simulink model "mat_acc"  (Simulink 8.7)
settings: Solver=VariableStepDiscrete  StartTime=0.0  StopTime=Accelerator_A10_param.endTime  MaxStep=1  RelTol=1e-3
PreLoadFcn:
  | % Run the setup script when the model is opened
  | setup_mat_acc;
InitFcn:
  | % Run the setup script again just before the
  | % model is run, so that any updates made
  | % after opening are applied.
  | setup_mat_acc;
undefined symbols (not defined in the file or in its folder): AdvDSPBChannelOutDisplay, dpoly, dspba_ChannelInVis, dspba_ChannelOutVis, dspba_internal_get_channel_ports, evalAionMaskParam, latency, primtype, value
libraries: DSPBAPrim x1114, DSPBAAvalonST x8, DSPBABase x5, DSPBAControl x2
(part 2 of 5)

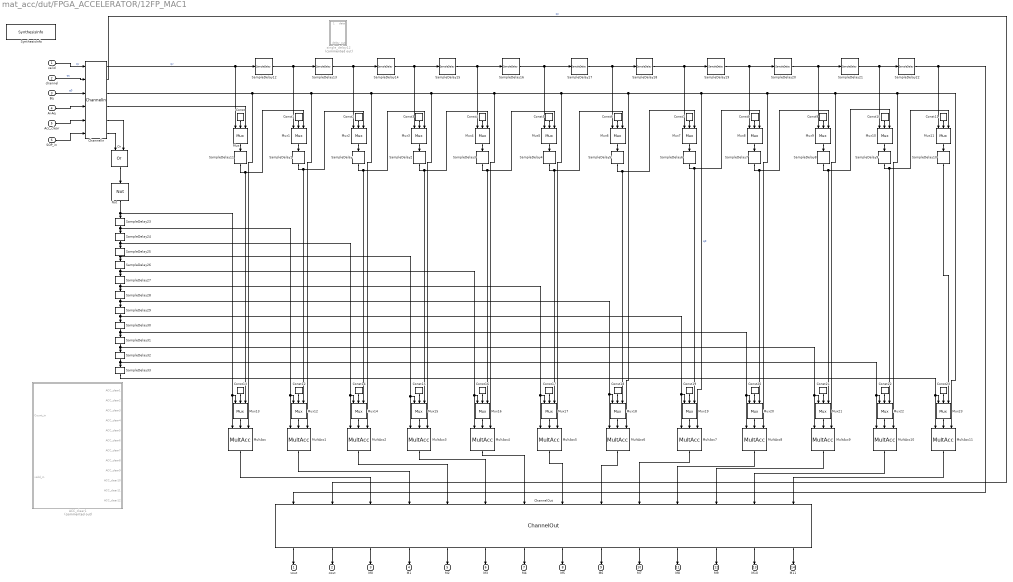
== system mat_acc/dut/FPGA_ACCELERATOR/12FP_MAC1 ==
  valid : Inport
  channel : Inport  Port=2
  Bq : Inport  Port=3
  Ai-Aq : Inport  Port=4
  Acc_clear : Inport  Port=5
  SOP_in : Inport  Port=6
  ACC_clear1 : Subsystem  Commented=on
  ChannelIn : DSPBAPrim/ChannelIn  primtype=channelin  nInputs=dspba_internal_get_channel_ports(gcb)  nOutputs=dspba_internal_get_channel_ports(gcb)  omode=Inherit via internal rule  otype=sfix(16)  scale=2^-15  rndmethod=Unbiased  factor=1  satmethod=Symmetric  shift_vec=[0 1 2 -1]  value=4  inPortNames=['v'; 'c'; '0'; '1'; '2'; '3'; '4'; '5'; '6'; '7'; '8'; '9'; 'A'; 'B'; 'D'; 'E'; 'F'; 'G'; 'H'; 'I'; 'J'; 'K'; 'L'; 'M'; 'N'; 'O'; 'P'; 'Q'; 'R'; 'S'; 'T'; 'U'; 'W'; 'X'; 'Y'; 'Z']  outPortNames=['v'; 'c'; '0'; '1'; '2'; '3'; '4'; '5'; '6'; '7'; '8'; '9'; 'A'; 'B'; 'D'; 'E'; 'F'; 'G'; 'H'; 'I'; 'J'; 'K'; 'L'; 'M'; 'N'; 'O'; 'P'; 'Q'; 'R'; 'S'; 'T'; 'U'; 'W'; 'X'; 'Y'; 'Z']  dspbaimage=dspba_prim.jpg  text=fprintf('In');  style=Optimised  dataSignals=4  foldingEnabled=off  channels=1  sampleRate=200  packetBeginPresent=off  packetBeginEnabled=off  visibilities=dspba_ChannelInVis(gcb)  latencyCorrection=0  version=20141013
  ChannelOut : DSPBAPrim/ChannelOut  primtype=channelout  nInputs=dspba_internal_get_channel_ports(gcb)  nOutputs=dspba_internal_get_channel_ports(gcb)  omode=Inherit via internal rule  otype=sfix(16)  scale=2^-15  rndmethod=Unbiased  factor=1  satmethod=Symmetric  shift_vec=[0 1 2 -1]  value=12  inPortNames=['v'; 'c'; '0'; '1'; '2'; '3'; '4'; '5'; '6'; '7'; '8'; '9'; 'A'; 'B'; 'D'; 'E'; 'F'; 'G'; 'H'; 'I'; 'J'; 'K'; 'L'; 'M'; 'N'; 'O'; 'P'; 'Q'; 'R'; 'S'; 'T'; 'U'; 'W'; 'X'; 'Y'; 'Z']  outPortNames=['v'; 'c'; '0'; '1'; '2'; '3'; '4'; '5'; '6'; '7'; '8'; '9'; 'A'; 'B'; 'D'; 'E'; 'F'; 'G'; 'H'; 'I'; 'J'; 'K'; 'L'; 'M'; 'N'; 'O'; 'P'; 'Q'; 'R'; 'S'; 'T'; 'U'; 'W'; 'X'; 'Y'; 'Z']  dspbaimage=dspba_prim.jpg  text=fprintf('Out%s', AdvDSPBChannelOutDisplay(latency));  style=Optimised  dataSignals=12  foldingEnabled=off  channels=1  sampleRate=200  packetBeginPresent=off  packetBeginEnabled=off  visibilities=dspba_ChannelOutVis(gcb)  latency=7  latencyCorrection=0  version=20141013
  Const{,1..23} (24 alike) : DSPBAPrim/Const  primtype=const  nInputs=0  nOutputs=1  omode=single  otype=sfix(16)  scale=2^-15  rndmethod=Unbiased  factor=1  satmethod=Symmetric  shift_vec=[0 1 2 -1]  value=0  inPortNames=['+'; '+';]  outPortNames=[' ']  dspbaimage=dspba_prim.jpg  text=fprintf('%s', num2str(value));  style=Optimised  visibilities=8 + 1024  floatPrecision=float32_m23  version=20120820
  MultAcc{,1..11} (12 alike) : DSPBAPrim/MultAcc  primtype=multaccfunc  nInputs=3  nOutputs=1  omode=Inherit via internal rule  otype=sfix(16)  scale=2^-15  rndmethod=Unbiased  factor=1  satmethod=Symmetric  shift_vec=[0 1 2 -1]  value=0  inPortNames="[ 'acc'; 'x  '; 'y  ']"  outPortNames=[]  dspbaimage=dspba_prim_float.jpg  text=disp('multAcc');  style=Optimised  visibilities=8+2^17  functionExpr=fpMultAcc  advOptions=[]  version=20121130
  Mux{,1..23} (24 alike) : DSPBAPrim/Mux  primtype=mux  nInputs=evalAionMaskParam(gcb,'value',1)+1  nOutputs=1  omode=Inherit via internal rule  otype=sfix(16)  scale=2^-15  rndmethod=Unbiased  factor=1  satmethod=Symmetric  shift_vec=[0 1 2 -1]  value=2  inPortNames=['s '; 'd0'; 'd1'; 'd2'; 'd3'; 'd4'; 'd5'; 'd6'; 'd7'; 'd8'; 'd9';]  outPortNames=[' ']  dspbaimage=dspba_prim.jpg  text=fprintf('%s', primtype);  style=Optimised  visibilities=1032  version=20131025
  Not : DSPBAPrim/Not  primtype=not  nInputs=1  nOutputs=1  omode=Inherit via internal rule  otype=sfix(16)  scale=2^-15  rndmethod=Unbiased  factor=1  satmethod=Symmetric  shift_vec=[0 1 2 -1]  value=0  inPortNames=[' '; ' ';]  outPortNames=[' ']  dspbaimage=dspba_prim.jpg  text=fprintf('~');  style=Optimised  visibilities=8  version=20090407
  Or : DSPBAPrim/Or  primtype=or  nInputs=2  nOutputs=1  omode=Inherit via internal rule  otype=sfix(16)  scale=2^-15  rndmethod=Unbiased  factor=1  satmethod=Symmetric  shift_vec=[0 1 2 -1]  value=0  inPortNames=[' '; ' '; ' '; ' '; ' '; ' '; ' '; ' '; ' '; ' '; ' '; ' '; ' '; ' '; ' '; ' '; ]  outPortNames=[' ']  dspbaimage=dspba_prim.jpg  text=fprintf('|');  style=Optimised  visibilities=8+2  version=20090407
  SampleDelay{,1..33} (34 alike) : DSPBAPrim/SampleDelay  primtype=sampdelay  nInputs=1  nOutputs=1  omode=Inherit via internal rule  otype=sfix(16)  scale=2^-15  rndmethod=Unbiased  factor=1  satmethod=Symmetric  shift_vec=[0 1 2 -1]  value=1  inPortNames=[' '; ' ';]  outPortNames=[' ']  dspbaimage=dspba_prim.jpg  text=dpoly(1, eye(1,value+1), 'z')  style=Optimised  visibilities=8 + 1024 + 2^17 + 2^18  flexible=off  slackgroup=0  augmented=0  version=20090407  advOptions=[]
  SynthesisInfo : DSPBAPrim/SynthesisInfo  primtype=synthinfo  nInputs=0  nOutputs=0  omode=Inherit via internal rule  otype=sfix(16)  scale=2^-15  rndmethod=Truncate  factor=1  satmethod=Symmetric  shift_vec=[0 1 2 -1]  value=99  inPortNames=[' '; ' ';]  outPortNames=[' ']  dspbaimage=dspba_prim_ctrl.jpg  text=fprintf('Style=%s', style);  style=Scheduled  visibilities=2^15+2^17+2^18+2^19  constraintInUse=on  constraintRelation==  constraintLimit=7  bitAccurate=off  version=20150220
  single_delay12 : Subsystem  Commented=on
  vout : Outport
  cout : Outport  Port=2
  M0 : Outport  Port=3
  M1 : Outport  Port=4
  M2 : Outport  Port=5
  M3 : Outport  Port=6
  M4 : Outport  Port=7
  M5 : Outport  Port=8
  M6 : Outport  Port=9
  M7 : Outport  Port=10
  M8 : Outport  Port=11
  M9 : Outport  Port=12
  M10 : Outport  Port=13
  M11 : Outport  Port=14
  wires:
  Mux23/1 -> MultAcc11/2
  Const23/1 -> Mux23/2
  Mux22/1 -> MultAcc10/2
  Const22/1 -> Mux22/2
  Mux21/1 -> MultAcc9/2
  Const21/1 -> Mux21/2
  Mux20/1 -> MultAcc8/2
  Const20/1 -> Mux20/2
  Mux19/1 -> MultAcc7/2
  Const19/1 -> Mux19/2
  Mux18/1 -> MultAcc6/2
  Const18/1 -> Mux18/2
  Mux17/1 -> MultAcc5/2
  Const17/1 -> Mux17/2
  Mux16/1 -> MultAcc4/2
  Const16/1 -> Mux16/2
  Mux15/1 -> MultAcc3/2
  Const15/1 -> Mux15/2
  Mux14/1 -> MultAcc2/2
  Const14/1 -> Mux14/2
  Mux12/1 -> MultAcc1/2
  Const12/1 -> Mux12/2
  Mux13/1 -> MultAcc/2
  Const13/1 -> Mux13/2
  Not/1 -> SampleDelay23/1, Mux13/1, MultAcc/1
  SampleDelay11/1 -> Mux1/3, Mux13/3
  Mux/1 -> SampleDelay11/1
  SampleDelay33/1 -> Mux23/1, MultAcc11/1
  SampleDelay32/1 -> SampleDelay33/1, MultAcc10/1, Mux22/1
  SampleDelay31/1 -> SampleDelay32/1, Mux21/1, MultAcc9/1
  SampleDelay30/1 -> SampleDelay31/1, MultAcc8/1, Mux20/1
  SampleDelay29/1 -> SampleDelay30/1, Mux19/1, MultAcc7/1
  SampleDelay28/1 -> SampleDelay29/1, Mux18/1, MultAcc6/1
  SampleDelay27/1 -> SampleDelay28/1, Mux17/1, MultAcc5/1
  SampleDelay26/1 -> SampleDelay27/1, Mux16/1, MultAcc4/1
  SampleDelay25/1 -> SampleDelay26/1, Mux15/1, MultAcc3/1
  SampleDelay24/1 -> SampleDelay25/1, Mux14/1, MultAcc2/1
  SampleDelay23/1 -> SampleDelay24/1, MultAcc1/1, Mux12/1
  SampleDelay22/1 -> Mux11/1, ChannelOut/1
  SampleDelay21/1 -> Mux10/1, SampleDelay22/1
  SampleDelay20/1 -> Mux9/1, SampleDelay21/1
  SampleDelay19/1 -> Mux8/1, SampleDelay20/1
  SampleDelay18/1 -> Mux7/1, SampleDelay19/1
  SampleDelay17/1 -> Mux6/1, SampleDelay18/1
  SampleDelay16/1 -> Mux5/1, SampleDelay17/1
  SampleDelay15/1 -> Mux4/1, SampleDelay16/1
  SampleDelay14/1 -> Mux3/1, SampleDelay15/1
  SampleDelay13/1 -> Mux2/1, SampleDelay14/1
  SampleDelay12/1 -> Mux1/1, SampleDelay13/1
  ChannelIn/6 -> Or/1
  SOP_in/1 -> ChannelIn/6
  ChannelIn/5 -> Or/2
  ChannelIn/1 -> Mux/1, SampleDelay12/1  "qv"
  SampleDelay10/1 -> Mux23/3
  SampleDelay9/1 -> Mux11/3, Mux22/3
  SampleDelay8/1 -> Mux10/3, Mux21/3
  SampleDelay7/1 -> Mux9/3, Mux20/3
  SampleDelay6/1 -> Mux8/3, Mux19/3
  SampleDelay5/1 -> Mux7/3, Mux18/3
  SampleDelay4/1 -> Mux6/3, Mux17/3
  SampleDelay3/1 -> Mux5/3, Mux16/3
  SampleDelay2/1 -> Mux4/3, Mux15/3
  SampleDelay1/1 -> Mux2/3, Mux12/3
  SampleDelay/1 -> Mux3/3, Mux14/3
  Const11/1 -> Mux11/2
  Const10/1 -> Mux10/2
  Const9/1 -> Mux9/2
  Const8/1 -> Mux8/2
  Const7/1 -> Mux7/2
  Const6/1 -> Mux6/2
  Const5/1 -> Mux5/2
  Const4/1 -> Mux4/2
  Const3/1 -> Mux3/2
  Const2/1 -> Mux2/2
  Const1/1 -> Mux1/2
  Const/1 -> Mux/2
  ChannelIn/2 -> ChannelOut/2  "qc"
  MultAcc11/1 -> ChannelOut/14
  MultAcc10/1 -> ChannelOut/13
  MultAcc9/1 -> ChannelOut/12
  MultAcc8/1 -> ChannelOut/11
  MultAcc7/1 -> ChannelOut/10
  MultAcc6/1 -> ChannelOut/9
  MultAcc5/1 -> ChannelOut/8
  MultAcc4/1 -> ChannelOut/7
  MultAcc3/1 -> ChannelOut/6
  MultAcc2/1 -> ChannelOut/5
  MultAcc1/1 -> ChannelOut/4
  MultAcc/1 -> ChannelOut/3
  ChannelOut/14 -> M11/1
  ChannelOut/13 -> M10/1
  ChannelOut/12 -> M9/1
  ChannelOut/11 -> M8/1
  ChannelOut/10 -> M7/1
  ChannelOut/9 -> M6/1
  ChannelOut/8 -> M5/1
  ChannelOut/7 -> M4/1
  ChannelOut/6 -> M3/1
  ChannelOut/5 -> M2/1
  ChannelOut/4 -> M1/1
  ChannelOut/3 -> M0/1
  ChannelOut/2 -> cout/1
  ChannelOut/1 -> vout/1
  Acc_clear/1 -> ChannelIn/5
  Ai-Aq/1 -> ChannelIn/4
  Bq/1 -> ChannelIn/3  "q0"
  channel/1 -> ChannelIn/2  "qc"
  valid/1 -> ChannelIn/1  "qv"
  Or/1 -> Not/1
  ChannelIn/4 -> Mux/3
  ChannelIn/3 -> MultAcc/3, MultAcc1/3, MultAcc2/3, MultAcc3/3, MultAcc4/3, MultAcc5/3, MultAcc6/3, MultAcc7/3, MultAcc8/3, MultAcc9/3, MultAcc10/3, MultAcc11/3  "q0"
  Mux1/1 -> SampleDelay1/1
  Mux2/1 -> SampleDelay/1
  Mux3/1 -> SampleDelay2/1
  Mux4/1 -> SampleDelay3/1
  Mux5/1 -> SampleDelay4/1
  Mux6/1 -> SampleDelay5/1
  Mux7/1 -> SampleDelay6/1
  Mux8/1 -> SampleDelay7/1
  Mux9/1 -> SampleDelay8/1
  Mux10/1 -> SampleDelay9/1
  Mux11/1 -> SampleDelay10/1

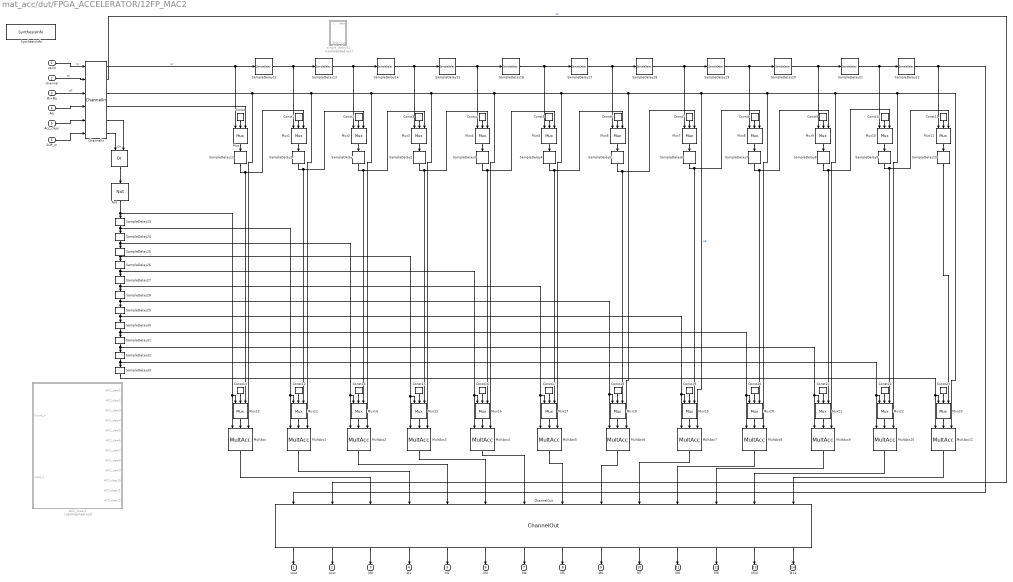
== system mat_acc/dut/FPGA_ACCELERATOR/12FP_MAC2 ==
  valid : Inport
  channel : Inport  Port=2
  Bi+Bq : Inport  Port=3
  Aq : Inport  Port=4
  Acc_clear : Inport  Port=5
  SOP_in : Inport  Port=6
  ACC_clear1 : Subsystem  Commented=on
  ChannelIn : DSPBAPrim/ChannelIn  primtype=channelin  nInputs=dspba_internal_get_channel_ports(gcb)  nOutputs=dspba_internal_get_channel_ports(gcb)  omode=Inherit via internal rule  otype=sfix(16)  scale=2^-15  rndmethod=Unbiased  factor=1  satmethod=Symmetric  shift_vec=[0 1 2 -1]  value=4  inPortNames=['v'; 'c'; '0'; '1'; '2'; '3'; '4'; '5'; '6'; '7'; '8'; '9'; 'A'; 'B'; 'D'; 'E'; 'F'; 'G'; 'H'; 'I'; 'J'; 'K'; 'L'; 'M'; 'N'; 'O'; 'P'; 'Q'; 'R'; 'S'; 'T'; 'U'; 'W'; 'X'; 'Y'; 'Z']  outPortNames=['v'; 'c'; '0'; '1'; '2'; '3'; '4'; '5'; '6'; '7'; '8'; '9'; 'A'; 'B'; 'D'; 'E'; 'F'; 'G'; 'H'; 'I'; 'J'; 'K'; 'L'; 'M'; 'N'; 'O'; 'P'; 'Q'; 'R'; 'S'; 'T'; 'U'; 'W'; 'X'; 'Y'; 'Z']  dspbaimage=dspba_prim.jpg  text=fprintf('In');  style=Optimised  dataSignals=4  foldingEnabled=off  channels=1  sampleRate=200  packetBeginPresent=off  packetBeginEnabled=off  visibilities=dspba_ChannelInVis(gcb)  latencyCorrection=0  version=20141013
  ChannelOut : DSPBAPrim/ChannelOut  primtype=channelout  nInputs=dspba_internal_get_channel_ports(gcb)  nOutputs=dspba_internal_get_channel_ports(gcb)  omode=Inherit via internal rule  otype=sfix(16)  scale=2^-15  rndmethod=Unbiased  factor=1  satmethod=Symmetric  shift_vec=[0 1 2 -1]  value=12  inPortNames=['v'; 'c'; '0'; '1'; '2'; '3'; '4'; '5'; '6'; '7'; '8'; '9'; 'A'; 'B'; 'D'; 'E'; 'F'; 'G'; 'H'; 'I'; 'J'; 'K'; 'L'; 'M'; 'N'; 'O'; 'P'; 'Q'; 'R'; 'S'; 'T'; 'U'; 'W'; 'X'; 'Y'; 'Z']  outPortNames=['v'; 'c'; '0'; '1'; '2'; '3'; '4'; '5'; '6'; '7'; '8'; '9'; 'A'; 'B'; 'D'; 'E'; 'F'; 'G'; 'H'; 'I'; 'J'; 'K'; 'L'; 'M'; 'N'; 'O'; 'P'; 'Q'; 'R'; 'S'; 'T'; 'U'; 'W'; 'X'; 'Y'; 'Z']  dspbaimage=dspba_prim.jpg  text=fprintf('Out%s', AdvDSPBChannelOutDisplay(latency));  style=Optimised  dataSignals=12  foldingEnabled=off  channels=1  sampleRate=200  packetBeginPresent=off  packetBeginEnabled=off  visibilities=dspba_ChannelOutVis(gcb)  latency=7  latencyCorrection=0  version=20141013
  Const{,1..23} (24 alike) : DSPBAPrim/Const  primtype=const  nInputs=0  nOutputs=1  omode=single  otype=sfix(16)  scale=2^-15  rndmethod=Unbiased  factor=1  satmethod=Symmetric  shift_vec=[0 1 2 -1]  value=0  inPortNames=['+'; '+';]  outPortNames=[' ']  dspbaimage=dspba_prim.jpg  text=fprintf('%s', num2str(value));  style=Optimised  visibilities=8 + 1024  floatPrecision=float32_m23  version=20120820
  MultAcc{,1..11} (12 alike) : DSPBAPrim/MultAcc  primtype=multaccfunc  nInputs=3  nOutputs=1  omode=Inherit via internal rule  otype=sfix(16)  scale=2^-15  rndmethod=Unbiased  factor=1  satmethod=Symmetric  shift_vec=[0 1 2 -1]  value=0  inPortNames="[ 'acc'; 'x  '; 'y  ']"  outPortNames=[]  dspbaimage=dspba_prim_float.jpg  text=disp('multAcc');  style=Optimised  visibilities=8+2^17  functionExpr=fpMultAcc  advOptions=[]  version=20121130
  Mux{,1..23} (24 alike) : DSPBAPrim/Mux  primtype=mux  nInputs=evalAionMaskParam(gcb,'value',1)+1  nOutputs=1  omode=Inherit via internal rule  otype=sfix(16)  scale=2^-15  rndmethod=Unbiased  factor=1  satmethod=Symmetric  shift_vec=[0 1 2 -1]  value=2  inPortNames=['s '; 'd0'; 'd1'; 'd2'; 'd3'; 'd4'; 'd5'; 'd6'; 'd7'; 'd8'; 'd9';]  outPortNames=[' ']  dspbaimage=dspba_prim.jpg  text=fprintf('%s', primtype);  style=Optimised  visibilities=1032  version=20131025
  Not : DSPBAPrim/Not  primtype=not  nInputs=1  nOutputs=1  omode=Inherit via internal rule  otype=sfix(16)  scale=2^-15  rndmethod=Unbiased  factor=1  satmethod=Symmetric  shift_vec=[0 1 2 -1]  value=0  inPortNames=[' '; ' ';]  outPortNames=[' ']  dspbaimage=dspba_prim.jpg  text=fprintf('~');  style=Optimised  visibilities=8  version=20090407
  Or : DSPBAPrim/Or  primtype=or  nInputs=2  nOutputs=1  omode=Inherit via internal rule  otype=sfix(16)  scale=2^-15  rndmethod=Unbiased  factor=1  satmethod=Symmetric  shift_vec=[0 1 2 -1]  value=0  inPortNames=[' '; ' '; ' '; ' '; ' '; ' '; ' '; ' '; ' '; ' '; ' '; ' '; ' '; ' '; ' '; ' '; ]  outPortNames=[' ']  dspbaimage=dspba_prim.jpg  text=fprintf('|');  style=Optimised  visibilities=8+2  version=20090407
  SampleDelay{,1..33} (34 alike) : DSPBAPrim/SampleDelay  primtype=sampdelay  nInputs=1  nOutputs=1  omode=Inherit via internal rule  otype=sfix(16)  scale=2^-15  rndmethod=Unbiased  factor=1  satmethod=Symmetric  shift_vec=[0 1 2 -1]  value=1  inPortNames=[' '; ' ';]  outPortNames=[' ']  dspbaimage=dspba_prim.jpg  text=dpoly(1, eye(1,value+1), 'z')  style=Optimised  visibilities=8 + 1024 + 2^17 + 2^18  flexible=off  slackgroup=0  augmented=0  version=20090407  advOptions=[]
  SynthesisInfo : DSPBAPrim/SynthesisInfo  primtype=synthinfo  nInputs=0  nOutputs=0  omode=Inherit via internal rule  otype=sfix(16)  scale=2^-15  rndmethod=Truncate  factor=1  satmethod=Symmetric  shift_vec=[0 1 2 -1]  value=99  inPortNames=[' '; ' ';]  outPortNames=[' ']  dspbaimage=dspba_prim_ctrl.jpg  text=fprintf('Style=%s', style);  style=Scheduled  visibilities=2^15+2^17+2^18+2^19  constraintInUse=on  constraintRelation==  constraintLimit=7  bitAccurate=off  version=20150220
  single_delay12 : Subsystem  Commented=on
  vout : Outport
  cout : Outport  Port=2
  M0 : Outport  Port=3
  M1 : Outport  Port=4
  M2 : Outport  Port=5
  M3 : Outport  Port=6
  M4 : Outport  Port=7
  M5 : Outport  Port=8
  M6 : Outport  Port=9
  M7 : Outport  Port=10
  M8 : Outport  Port=11
  M9 : Outport  Port=12
  M10 : Outport  Port=13
  M11 : Outport  Port=14
  wires:
  Mux11/1 -> SampleDelay10/1
  Mux10/1 -> SampleDelay9/1
  Mux9/1 -> SampleDelay8/1
  Mux8/1 -> SampleDelay7/1
  Mux7/1 -> SampleDelay6/1
  Mux6/1 -> SampleDelay5/1
  Mux5/1 -> SampleDelay4/1
  Mux4/1 -> SampleDelay3/1
  Mux3/1 -> SampleDelay2/1
  Mux2/1 -> SampleDelay/1
  Mux1/1 -> SampleDelay1/1
  ChannelIn/3 -> MultAcc11/3, MultAcc10/3, MultAcc9/3, MultAcc8/3, MultAcc7/3, MultAcc6/3, MultAcc5/3, MultAcc4/3, MultAcc3/3, MultAcc2/3, MultAcc1/3, MultAcc/3  "q0"
  ChannelIn/4 -> Mux/3
  Or/1 -> Not/1
  valid/1 -> ChannelIn/1  "qv"
  channel/1 -> ChannelIn/2  "qc"
  Bi+Bq/1 -> ChannelIn/3  "q0"
  Aq/1 -> ChannelIn/4
  Acc_clear/1 -> ChannelIn/5
  ChannelOut/1 -> vout/1
  ChannelOut/2 -> cout/1
  ChannelOut/3 -> M0/1
  ChannelOut/4 -> M1/1
  ChannelOut/5 -> M2/1
  ChannelOut/6 -> M3/1
  ChannelOut/7 -> M4/1
  ChannelOut/8 -> M5/1
  ChannelOut/9 -> M6/1
  ChannelOut/10 -> M7/1
  ChannelOut/11 -> M8/1
  ChannelOut/12 -> M9/1
  ChannelOut/13 -> M10/1
  ChannelOut/14 -> M11/1
  MultAcc/1 -> ChannelOut/3
  MultAcc1/1 -> ChannelOut/4
  MultAcc2/1 -> ChannelOut/5
  MultAcc3/1 -> ChannelOut/6
  MultAcc4/1 -> ChannelOut/7
  MultAcc5/1 -> ChannelOut/8
  MultAcc6/1 -> ChannelOut/9
  MultAcc7/1 -> ChannelOut/10
  MultAcc8/1 -> ChannelOut/11
  MultAcc9/1 -> ChannelOut/12
  MultAcc10/1 -> ChannelOut/13
  MultAcc11/1 -> ChannelOut/14
  ChannelIn/2 -> ChannelOut/2  "qc"
  Const/1 -> Mux/2
  Const1/1 -> Mux1/2
  Const2/1 -> Mux2/2
  Const3/1 -> Mux3/2
  Const4/1 -> Mux4/2
  Const5/1 -> Mux5/2
  Const6/1 -> Mux6/2
  Const7/1 -> Mux7/2
  Const8/1 -> Mux8/2
  Const9/1 -> Mux9/2
  Const10/1 -> Mux10/2
  Const11/1 -> Mux11/2
  SampleDelay/1 -> Mux14/3, Mux3/3
  SampleDelay1/1 -> Mux12/3, Mux2/3
  SampleDelay2/1 -> Mux15/3, Mux4/3
  SampleDelay3/1 -> Mux16/3, Mux5/3
  SampleDelay4/1 -> Mux17/3, Mux6/3
  SampleDelay5/1 -> Mux18/3, Mux7/3
  SampleDelay6/1 -> Mux19/3, Mux8/3
  SampleDelay7/1 -> Mux20/3, Mux9/3
  SampleDelay8/1 -> Mux21/3, Mux10/3
  SampleDelay9/1 -> Mux22/3, Mux11/3
  SampleDelay10/1 -> Mux23/3
  ChannelIn/1 -> SampleDelay12/1, Mux/1  "qv"
  ChannelIn/5 -> Or/2
  SOP_in/1 -> ChannelIn/6
  ChannelIn/6 -> Or/1
  SampleDelay12/1 -> SampleDelay13/1, Mux1/1
  SampleDelay13/1 -> SampleDelay14/1, Mux2/1
  SampleDelay14/1 -> SampleDelay15/1, Mux3/1
  SampleDelay15/1 -> SampleDelay16/1, Mux4/1
  SampleDelay16/1 -> SampleDelay17/1, Mux5/1
  SampleDelay17/1 -> SampleDelay18/1, Mux6/1
  SampleDelay18/1 -> SampleDelay19/1, Mux7/1
  SampleDelay19/1 -> SampleDelay20/1, Mux8/1
  SampleDelay20/1 -> SampleDelay21/1, Mux9/1
  SampleDelay21/1 -> SampleDelay22/1, Mux10/1
  SampleDelay22/1 -> ChannelOut/1, Mux11/1
  SampleDelay23/1 -> Mux12/1, MultAcc1/1, SampleDelay24/1
  SampleDelay24/1 -> MultAcc2/1, Mux14/1, SampleDelay25/1
  SampleDelay25/1 -> MultAcc3/1, Mux15/1, SampleDelay26/1
  SampleDelay26/1 -> MultAcc4/1, Mux16/1, SampleDelay27/1
  SampleDelay27/1 -> MultAcc5/1, Mux17/1, SampleDelay28/1
  SampleDelay28/1 -> MultAcc6/1, Mux18/1, SampleDelay29/1
  SampleDelay29/1 -> MultAcc7/1, Mux19/1, SampleDelay30/1
  SampleDelay30/1 -> Mux20/1, MultAcc8/1, SampleDelay31/1
  SampleDelay31/1 -> MultAcc9/1, Mux21/1, SampleDelay32/1
  SampleDelay32/1 -> Mux22/1, MultAcc10/1, SampleDelay33/1
  SampleDelay33/1 -> MultAcc11/1, Mux23/1
  Mux/1 -> SampleDelay11/1
  SampleDelay11/1 -> Mux13/3, Mux1/3
  Not/1 -> MultAcc/1, Mux13/1, SampleDelay23/1
  Const13/1 -> Mux13/2
  Mux13/1 -> MultAcc/2
  Const12/1 -> Mux12/2
  Mux12/1 -> MultAcc1/2
  Const14/1 -> Mux14/2
  Mux14/1 -> MultAcc2/2
  Const15/1 -> Mux15/2
  Mux15/1 -> MultAcc3/2
  Const16/1 -> Mux16/2
  Mux16/1 -> MultAcc4/2
  Const17/1 -> Mux17/2
  Mux17/1 -> MultAcc5/2
  Const18/1 -> Mux18/2
  Mux18/1 -> MultAcc6/2
  Const19/1 -> Mux19/2
  Mux19/1 -> MultAcc7/2
  Const20/1 -> Mux20/2
  Mux20/1 -> MultAcc8/2
  Const21/1 -> Mux21/2
  Mux21/1 -> MultAcc9/2
  Const22/1 -> Mux22/2
  Mux22/1 -> MultAcc10/2
  Const23/1 -> Mux23/2
  Mux23/1 -> MultAcc11/2

== system mat_acc/dut/FPGA_ACCELERATOR/12FP_MUX ==
  Valid : Inport
  Channel : Inport  Port=2
  I0 : Inport  Port=3
  I1 : Inport  Port=4
  I2 : Inport  Port=5
  I3 : Inport  Port=6
  I4 : Inport  Port=7
  I5 : Inport  Port=8
  I6 : Inport  Port=9
  I7 : Inport  Port=10
  I8 : Inport  Port=11
  I9 : Inport  Port=12
  I10 : Inport  Port=13
  I11 : Inport  Port=14
  MUX_select : Inport  Port=15
  ChannelIn : DSPBAPrim/ChannelIn  primtype=channelin  nInputs=dspba_internal_get_channel_ports(gcb)  nOutputs=dspba_internal_get_channel_ports(gcb)  omode=Inherit via internal rule  otype=sfix(16)  scale=2^-15  rndmethod=Unbiased  factor=1  satmethod=Symmetric  shift_vec=[0 1 2 -1]  value=13  inPortNames=['v'; 'c'; '0'; '1'; '2'; '3'; '4'; '5'; '6'; '7'; '8'; '9'; 'A'; 'B'; 'D'; 'E'; 'F'; 'G'; 'H'; 'I'; 'J'; 'K'; 'L'; 'M'; 'N'; 'O'; 'P'; 'Q'; 'R'; 'S'; 'T'; 'U'; 'W'; 'X'; 'Y'; 'Z']  outPortNames=['v'; 'c'; '0'; '1'; '2'; '3'; '4'; '5'; '6'; '7'; '8'; '9'; 'A'; 'B'; 'D'; 'E'; 'F'; 'G'; 'H'; 'I'; 'J'; 'K'; 'L'; 'M'; 'N'; 'O'; 'P'; 'Q'; 'R'; 'S'; 'T'; 'U'; 'W'; 'X'; 'Y'; 'Z']  dspbaimage=dspba_prim.jpg  text=fprintf('In');  style=Optimised  dataSignals=13  foldingEnabled=off  channels=1  sampleRate=200  packetBeginPresent=off  packetBeginEnabled=off  visibilities=dspba_ChannelInVis(gcb)  latencyCorrection=0  version=20141013
  ChannelOut : DSPBAPrim/ChannelOut  primtype=channelout  nInputs=dspba_internal_get_channel_ports(gcb)  nOutputs=dspba_internal_get_channel_ports(gcb)  omode=Inherit via internal rule  otype=sfix(16)  scale=2^-15  rndmethod=Unbiased  factor=1  satmethod=Symmetric  shift_vec=[0 1 2 -1]  value=1  inPortNames=['v'; 'c'; '0'; '1'; '2'; '3'; '4'; '5'; '6'; '7'; '8'; '9'; 'A'; 'B'; 'D'; 'E'; 'F'; 'G'; 'H'; 'I'; 'J'; 'K'; 'L'; 'M'; 'N'; 'O'; 'P'; 'Q'; 'R'; 'S'; 'T'; 'U'; 'W'; 'X'; 'Y'; 'Z']  outPortNames=['v'; 'c'; '0'; '1'; '2'; '3'; '4'; '5'; '6'; '7'; '8'; '9'; 'A'; 'B'; 'D'; 'E'; 'F'; 'G'; 'H'; 'I'; 'J'; 'K'; 'L'; 'M'; 'N'; 'O'; 'P'; 'Q'; 'R'; 'S'; 'T'; 'U'; 'W'; 'X'; 'Y'; 'Z']  dspbaimage=dspba_prim.jpg  text=fprintf('Out%s', AdvDSPBChannelOutDisplay(latency));  style=Optimised  dataSignals=1  foldingEnabled=off  channels=1  sampleRate=200  packetBeginPresent=off  packetBeginEnabled=off  visibilities=dspba_ChannelOutVis(gcb)  latency=2  latencyCorrection=0  version=20141013
  Const : DSPBAPrim/Const  primtype=const  nInputs=0  nOutputs=1  omode=single  otype=sfix(16)  scale=2^-15  rndmethod=Unbiased  factor=1  satmethod=Symmetric  shift_vec=[0 1 2 -1]  value=0  inPortNames=['+'; '+';]  outPortNames=[' ']  dspbaimage=dspba_prim.jpg  text=fprintf('%s', num2str(value));  style=Optimised  visibilities=8 + 1024  floatPrecision=float32_m23  version=20120820
  Mux real : DSPBAPrim/Mux  primtype=mux  nInputs=evalAionMaskParam(gcb,'value',1)+1  nOutputs=1  omode=Inherit via internal rule  otype=sfix(16)  scale=2^-15  rndmethod=Unbiased  factor=1  satmethod=Symmetric  shift_vec=[0 1 2 -1]  value=13  inPortNames=['s '; 'd0'; 'd1'; 'd2'; 'd3'; 'd4'; 'd5'; 'd6'; 'd7'; 'd8'; 'd9';]  outPortNames=[' ']  dspbaimage=dspba_prim.jpg  text=fprintf('%s', primtype);  style=Optimised  visibilities=1032  version=20131025
  SampleDelay : DSPBAPrim/SampleDelay  primtype=sampdelay  nInputs=1  nOutputs=1  omode=Inherit via internal rule  otype=sfix(16)  scale=2^-15  rndmethod=Unbiased  factor=1  satmethod=Symmetric  shift_vec=[0 1 2 -1]  value=5  inPortNames=[' '; ' ';]  outPortNames=[' ']  dspbaimage=dspba_prim.jpg  text=dpoly(1, eye(1,value+1), 'z')  style=Optimised  visibilities=8 + 1024 + 2^17 + 2^18  flexible=off  slackgroup=0  augmented=0  version=20090407  advOptions=[]
  SynthesisInfo : DSPBAPrim/SynthesisInfo  primtype=synthinfo  nInputs=0  nOutputs=0  omode=Inherit via internal rule  otype=sfix(16)  scale=2^-15  rndmethod=Truncate  factor=1  satmethod=Symmetric  shift_vec=[0 1 2 -1]  value=99  inPortNames=[' '; ' ';]  outPortNames=[' ']  dspbaimage=dspba_prim_ctrl.jpg  text=fprintf('Style=%s', style);  style=Scheduled  visibilities=2^15+2^17+2^18+2^19  constraintInUse=on  constraintRelation==  constraintLimit=2  bitAccurate=off  version=20150220
  vout : Outport
  cout : Outport  Port=2
  (Bi-Bq)*Ai : Outport  Port=3
  wires:
  ChannelIn/14 -> Mux real/14
  ChannelIn/13 -> Mux real/13
  ChannelIn/12 -> Mux real/12
  ChannelIn/11 -> Mux real/11
  ChannelIn/10 -> Mux real/10
  ChannelIn/9 -> Mux real/9
  ChannelIn/8 -> Mux real/8
  ChannelIn/7 -> Mux real/7
  ChannelIn/6 -> Mux real/6
  ChannelIn/5 -> Mux real/5
  ChannelIn/4 -> Mux real/4
  ChannelIn/3 -> Mux real/3
  ChannelIn/15 -> SampleDelay/1
  ChannelIn/2 -> ChannelOut/2
  Mux real/1 -> ChannelOut/3
  Const/1 -> Mux real/2
  Valid/1 -> ChannelIn/1
  Channel/1 -> ChannelIn/2
  I0/1 -> ChannelIn/3
  I1/1 -> ChannelIn/4
  I2/1 -> ChannelIn/5
  I3/1 -> ChannelIn/6
  I4/1 -> ChannelIn/7
  I5/1 -> ChannelIn/8
  I6/1 -> ChannelIn/9
  I7/1 -> ChannelIn/10
  I8/1 -> ChannelIn/11
  I9/1 -> ChannelIn/12
  I10/1 -> ChannelIn/13
  I11/1 -> ChannelIn/14
  MUX_select/1 -> ChannelIn/15
  ChannelOut/1 -> vout/1
  ChannelOut/2 -> cout/1
  ChannelOut/3 -> (Bi-Bq)*Ai/1
  SampleDelay/1 -> Mux real/1
  ChannelIn/1 -> ChannelOut/1

== system mat_acc/dut/FPGA_ACCELERATOR/12FP_MUX1 ==
  Valid : Inport
  Channel : Inport  Port=2
  I0 : Inport  Port=3
  I1 : Inport  Port=4
  I2 : Inport  Port=5
  I3 : Inport  Port=6
  I4 : Inport  Port=7
  I5 : Inport  Port=8
  I6 : Inport  Port=9
  I7 : Inport  Port=10
  I8 : Inport  Port=11
  I9 : Inport  Port=12
  I10 : Inport  Port=13
  I11 : Inport  Port=14
  MUX_select : Inport  Port=15
  ChannelIn : DSPBAPrim/ChannelIn  primtype=channelin  nInputs=dspba_internal_get_channel_ports(gcb)  nOutputs=dspba_internal_get_channel_ports(gcb)  omode=Inherit via internal rule  otype=sfix(16)  scale=2^-15  rndmethod=Unbiased  factor=1  satmethod=Symmetric  shift_vec=[0 1 2 -1]  value=13  inPortNames=['v'; 'c'; '0'; '1'; '2'; '3'; '4'; '5'; '6'; '7'; '8'; '9'; 'A'; 'B'; 'D'; 'E'; 'F'; 'G'; 'H'; 'I'; 'J'; 'K'; 'L'; 'M'; 'N'; 'O'; 'P'; 'Q'; 'R'; 'S'; 'T'; 'U'; 'W'; 'X'; 'Y'; 'Z']  outPortNames=['v'; 'c'; '0'; '1'; '2'; '3'; '4'; '5'; '6'; '7'; '8'; '9'; 'A'; 'B'; 'D'; 'E'; 'F'; 'G'; 'H'; 'I'; 'J'; 'K'; 'L'; 'M'; 'N'; 'O'; 'P'; 'Q'; 'R'; 'S'; 'T'; 'U'; 'W'; 'X'; 'Y'; 'Z']  dspbaimage=dspba_prim.jpg  text=fprintf('In');  style=Optimised  dataSignals=13  foldingEnabled=off  channels=1  sampleRate=200  packetBeginPresent=off  packetBeginEnabled=off  visibilities=dspba_ChannelInVis(gcb)  latencyCorrection=0  version=20141013
  ChannelOut : DSPBAPrim/ChannelOut  primtype=channelout  nInputs=dspba_internal_get_channel_ports(gcb)  nOutputs=dspba_internal_get_channel_ports(gcb)  omode=Inherit via internal rule  otype=sfix(16)  scale=2^-15  rndmethod=Unbiased  factor=1  satmethod=Symmetric  shift_vec=[0 1 2 -1]  value=1  inPortNames=['v'; 'c'; '0'; '1'; '2'; '3'; '4'; '5'; '6'; '7'; '8'; '9'; 'A'; 'B'; 'D'; 'E'; 'F'; 'G'; 'H'; 'I'; 'J'; 'K'; 'L'; 'M'; 'N'; 'O'; 'P'; 'Q'; 'R'; 'S'; 'T'; 'U'; 'W'; 'X'; 'Y'; 'Z']  outPortNames=['v'; 'c'; '0'; '1'; '2'; '3'; '4'; '5'; '6'; '7'; '8'; '9'; 'A'; 'B'; 'D'; 'E'; 'F'; 'G'; 'H'; 'I'; 'J'; 'K'; 'L'; 'M'; 'N'; 'O'; 'P'; 'Q'; 'R'; 'S'; 'T'; 'U'; 'W'; 'X'; 'Y'; 'Z']  dspbaimage=dspba_prim.jpg  text=fprintf('Out%s', AdvDSPBChannelOutDisplay(latency));  style=Optimised  dataSignals=1  foldingEnabled=off  channels=1  sampleRate=200  packetBeginPresent=off  packetBeginEnabled=off  visibilities=dspba_ChannelOutVis(gcb)  latency=2  latencyCorrection=0  version=20141013
  Const : DSPBAPrim/Const  primtype=const  nInputs=0  nOutputs=1  omode=single  otype=sfix(16)  scale=2^-15  rndmethod=Unbiased  factor=1  satmethod=Symmetric  shift_vec=[0 1 2 -1]  value=0  inPortNames=['+'; '+';]  outPortNames=[' ']  dspbaimage=dspba_prim.jpg  text=fprintf('%s', num2str(value));  style=Optimised  visibilities=8 + 1024  floatPrecision=float32_m23  version=20120820
  Mux real : DSPBAPrim/Mux  primtype=mux  nInputs=evalAionMaskParam(gcb,'value',1)+1  nOutputs=1  omode=Inherit via internal rule  otype=sfix(16)  scale=2^-15  rndmethod=Unbiased  factor=1  satmethod=Symmetric  shift_vec=[0 1 2 -1]  value=13  inPortNames=['s '; 'd0'; 'd1'; 'd2'; 'd3'; 'd4'; 'd5'; 'd6'; 'd7'; 'd8'; 'd9';]  outPortNames=[' ']  dspbaimage=dspba_prim.jpg  text=fprintf('%s', primtype);  style=Optimised  visibilities=1032  version=20131025
  SampleDelay : DSPBAPrim/SampleDelay  primtype=sampdelay  nInputs=1  nOutputs=1  omode=Inherit via internal rule  otype=sfix(16)  scale=2^-15  rndmethod=Unbiased  factor=1  satmethod=Symmetric  shift_vec=[0 1 2 -1]  value=5  inPortNames=[' '; ' ';]  outPortNames=[' ']  dspbaimage=dspba_prim.jpg  text=dpoly(1, eye(1,value+1), 'z')  style=Optimised  visibilities=8 + 1024 + 2^17 + 2^18  flexible=off  slackgroup=0  augmented=0  version=20090407  advOptions=[]
  SynthesisInfo : DSPBAPrim/SynthesisInfo  primtype=synthinfo  nInputs=0  nOutputs=0  omode=Inherit via internal rule  otype=sfix(16)  scale=2^-15  rndmethod=Truncate  factor=1  satmethod=Symmetric  shift_vec=[0 1 2 -1]  value=99  inPortNames=[' '; ' ';]  outPortNames=[' ']  dspbaimage=dspba_prim_ctrl.jpg  text=fprintf('Style=%s', style);  style=Scheduled  visibilities=2^15+2^17+2^18+2^19  constraintInUse=on  constraintRelation==  constraintLimit=2  bitAccurate=off  version=20150220
  vout : Outport
  cout : Outport  Port=2
  Bq*(Ai-Aq) : Outport  Port=3
  wires:
  ChannelOut/3 -> Bq*(Ai-Aq)/1
  ChannelOut/2 -> cout/1
  ChannelOut/1 -> vout/1
  MUX_select/1 -> ChannelIn/15
  I11/1 -> ChannelIn/14
  I10/1 -> ChannelIn/13
  I9/1 -> ChannelIn/12
  I8/1 -> ChannelIn/11
  I7/1 -> ChannelIn/10
  I6/1 -> ChannelIn/9
  I5/1 -> ChannelIn/8
  I4/1 -> ChannelIn/7
  I3/1 -> ChannelIn/6
  I2/1 -> ChannelIn/5
  I1/1 -> ChannelIn/4
  I0/1 -> ChannelIn/3
  Channel/1 -> ChannelIn/2
  Valid/1 -> ChannelIn/1
  Const/1 -> Mux real/2
  Mux real/1 -> ChannelOut/3
  ChannelIn/2 -> ChannelOut/2
  ChannelIn/1 -> ChannelOut/1
  ChannelIn/15 -> SampleDelay/1
  ChannelIn/3 -> Mux real/3
  ChannelIn/4 -> Mux real/4
  ChannelIn/5 -> Mux real/5
  ChannelIn/6 -> Mux real/6
  ChannelIn/7 -> Mux real/7
  ChannelIn/8 -> Mux real/8
  ChannelIn/9 -> Mux real/9
  ChannelIn/10 -> Mux real/10
  ChannelIn/11 -> Mux real/11
  ChannelIn/12 -> Mux real/12
  ChannelIn/13 -> Mux real/13
  ChannelIn/14 -> Mux real/14
  SampleDelay/1 -> Mux real/1

== system mat_acc/dut/FPGA_ACCELERATOR/12FP_MUX2 ==
  Valid : Inport
  Channel : Inport  Port=2
  I0 : Inport  Port=3
  I1 : Inport  Port=4
  I2 : Inport  Port=5
  I3 : Inport  Port=6
  I4 : Inport  Port=7
  I5 : Inport  Port=8
  I6 : Inport  Port=9
  I7 : Inport  Port=10
  I8 : Inport  Port=11
  I9 : Inport  Port=12
  I10 : Inport  Port=13
  I11 : Inport  Port=14
  MUX_select : Inport  Port=15
  ChannelIn : DSPBAPrim/ChannelIn  primtype=channelin  nInputs=dspba_internal_get_channel_ports(gcb)  nOutputs=dspba_internal_get_channel_ports(gcb)  omode=Inherit via internal rule  otype=sfix(16)  scale=2^-15  rndmethod=Unbiased  factor=1  satmethod=Symmetric  shift_vec=[0 1 2 -1]  value=13  inPortNames=['v'; 'c'; '0'; '1'; '2'; '3'; '4'; '5'; '6'; '7'; '8'; '9'; 'A'; 'B'; 'D'; 'E'; 'F'; 'G'; 'H'; 'I'; 'J'; 'K'; 'L'; 'M'; 'N'; 'O'; 'P'; 'Q'; 'R'; 'S'; 'T'; 'U'; 'W'; 'X'; 'Y'; 'Z']  outPortNames=['v'; 'c'; '0'; '1'; '2'; '3'; '4'; '5'; '6'; '7'; '8'; '9'; 'A'; 'B'; 'D'; 'E'; 'F'; 'G'; 'H'; 'I'; 'J'; 'K'; 'L'; 'M'; 'N'; 'O'; 'P'; 'Q'; 'R'; 'S'; 'T'; 'U'; 'W'; 'X'; 'Y'; 'Z']  dspbaimage=dspba_prim.jpg  text=fprintf('In');  style=Optimised  dataSignals=13  foldingEnabled=off  channels=1  sampleRate=200  packetBeginPresent=off  packetBeginEnabled=off  visibilities=dspba_ChannelInVis(gcb)  latencyCorrection=0  version=20141013
  ChannelOut : DSPBAPrim/ChannelOut  primtype=channelout  nInputs=dspba_internal_get_channel_ports(gcb)  nOutputs=dspba_internal_get_channel_ports(gcb)  omode=Inherit via internal rule  otype=sfix(16)  scale=2^-15  rndmethod=Unbiased  factor=1  satmethod=Symmetric  shift_vec=[0 1 2 -1]  value=1  inPortNames=['v'; 'c'; '0'; '1'; '2'; '3'; '4'; '5'; '6'; '7'; '8'; '9'; 'A'; 'B'; 'D'; 'E'; 'F'; 'G'; 'H'; 'I'; 'J'; 'K'; 'L'; 'M'; 'N'; 'O'; 'P'; 'Q'; 'R'; 'S'; 'T'; 'U'; 'W'; 'X'; 'Y'; 'Z']  outPortNames=['v'; 'c'; '0'; '1'; '2'; '3'; '4'; '5'; '6'; '7'; '8'; '9'; 'A'; 'B'; 'D'; 'E'; 'F'; 'G'; 'H'; 'I'; 'J'; 'K'; 'L'; 'M'; 'N'; 'O'; 'P'; 'Q'; 'R'; 'S'; 'T'; 'U'; 'W'; 'X'; 'Y'; 'Z']  dspbaimage=dspba_prim.jpg  text=fprintf('Out%s', AdvDSPBChannelOutDisplay(latency));  style=Optimised  dataSignals=1  foldingEnabled=off  channels=1  sampleRate=200  packetBeginPresent=off  packetBeginEnabled=off  visibilities=dspba_ChannelOutVis(gcb)  latency=2  latencyCorrection=0  version=20141013
  Const : DSPBAPrim/Const  primtype=const  nInputs=0  nOutputs=1  omode=single  otype=sfix(16)  scale=2^-15  rndmethod=Unbiased  factor=1  satmethod=Symmetric  shift_vec=[0 1 2 -1]  value=0  inPortNames=['+'; '+';]  outPortNames=[' ']  dspbaimage=dspba_prim.jpg  text=fprintf('%s', num2str(value));  style=Optimised  visibilities=8 + 1024  floatPrecision=float32_m23  version=20120820
  Mux real : DSPBAPrim/Mux  primtype=mux  nInputs=evalAionMaskParam(gcb,'value',1)+1  nOutputs=1  omode=Inherit via internal rule  otype=sfix(16)  scale=2^-15  rndmethod=Unbiased  factor=1  satmethod=Symmetric  shift_vec=[0 1 2 -1]  value=13  inPortNames=['s '; 'd0'; 'd1'; 'd2'; 'd3'; 'd4'; 'd5'; 'd6'; 'd7'; 'd8'; 'd9';]  outPortNames=[' ']  dspbaimage=dspba_prim.jpg  text=fprintf('%s', primtype);  style=Optimised  visibilities=1032  version=20131025
  SampleDelay : DSPBAPrim/SampleDelay  primtype=sampdelay  nInputs=1  nOutputs=1  omode=Inherit via internal rule  otype=sfix(16)  scale=2^-15  rndmethod=Unbiased  factor=1  satmethod=Symmetric  shift_vec=[0 1 2 -1]  value=5  inPortNames=[' '; ' ';]  outPortNames=[' ']  dspbaimage=dspba_prim.jpg  text=dpoly(1, eye(1,value+1), 'z')  style=Optimised  visibilities=8 + 1024 + 2^17 + 2^18  flexible=off  slackgroup=0  augmented=0  version=20090407  advOptions=[]
  SynthesisInfo : DSPBAPrim/SynthesisInfo  primtype=synthinfo  nInputs=0  nOutputs=0  omode=Inherit via internal rule  otype=sfix(16)  scale=2^-15  rndmethod=Truncate  factor=1  satmethod=Symmetric  shift_vec=[0 1 2 -1]  value=99  inPortNames=[' '; ' ';]  outPortNames=[' ']  dspbaimage=dspba_prim_ctrl.jpg  text=fprintf('Style=%s', style);  style=Scheduled  visibilities=2^15+2^17+2^18+2^19  constraintInUse=on  constraintRelation==  constraintLimit=2  bitAccurate=off  version=20150220
  vout : Outport
  cout : Outport  Port=2
  (Bi+Bq)*Aq : Outport  Port=3
  wires:
  ChannelIn/14 -> Mux real/14
  ChannelIn/13 -> Mux real/13
  ChannelIn/12 -> Mux real/12
  ChannelIn/11 -> Mux real/11
  ChannelIn/10 -> Mux real/10
  ChannelIn/9 -> Mux real/9
  ChannelIn/8 -> Mux real/8
  ChannelIn/7 -> Mux real/7
  ChannelIn/6 -> Mux real/6
  ChannelIn/5 -> Mux real/5
  ChannelIn/4 -> Mux real/4
  ChannelIn/3 -> Mux real/3
  ChannelIn/15 -> SampleDelay/1
  ChannelIn/1 -> ChannelOut/1
  ChannelIn/2 -> ChannelOut/2
  Mux real/1 -> ChannelOut/3
  Const/1 -> Mux real/2
  Valid/1 -> ChannelIn/1
  Channel/1 -> ChannelIn/2
  I0/1 -> ChannelIn/3
  I1/1 -> ChannelIn/4
  I2/1 -> ChannelIn/5
  I3/1 -> ChannelIn/6
  I4/1 -> ChannelIn/7
  I5/1 -> ChannelIn/8
  I6/1 -> ChannelIn/9
  I7/1 -> ChannelIn/10
  I8/1 -> ChannelIn/11
  I9/1 -> ChannelIn/12
  I10/1 -> ChannelIn/13
  I11/1 -> ChannelIn/14
  MUX_select/1 -> ChannelIn/15
  ChannelOut/1 -> vout/1
  ChannelOut/2 -> cout/1
  ChannelOut/3 -> (Bi+Bq)*Aq/1
  SampleDelay/1 -> Mux real/1

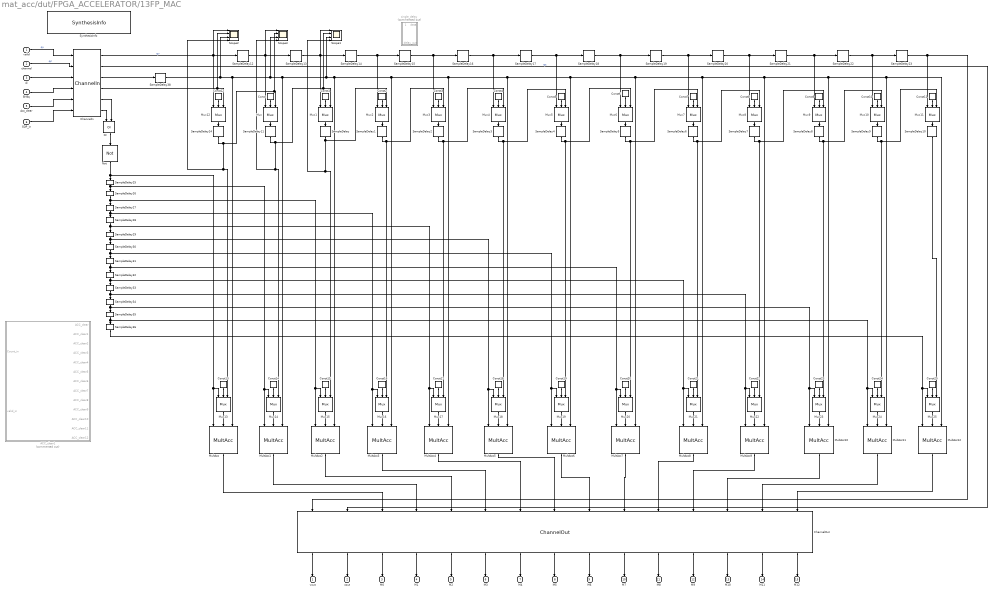
== system mat_acc/dut/FPGA_ACCELERATOR/13FP_MAC ==
  valid : Inport
  channel : Inport  Port=2
  Ai : Inport  Port=3
  Bi-Bq : Inport  Port=4
  Acc_clear : Inport  Port=5
  SOP_in : Inport  Port=6
  ACC_clear1 : Subsystem  Commented=on
  ChannelIn : DSPBAPrim/ChannelIn  primtype=channelin  nInputs=dspba_internal_get_channel_ports(gcb)  nOutputs=dspba_internal_get_channel_ports(gcb)  omode=Inherit via internal rule  otype=sfix(16)  scale=2^-15  rndmethod=Unbiased  factor=1  satmethod=Symmetric  shift_vec=[0 1 2 -1]  value=4  inPortNames=['v'; 'c'; '0'; '1'; '2'; '3'; '4'; '5'; '6'; '7'; '8'; '9'; 'A'; 'B'; 'D'; 'E'; 'F'; 'G'; 'H'; 'I'; 'J'; 'K'; 'L'; 'M'; 'N'; 'O'; 'P'; 'Q'; 'R'; 'S'; 'T'; 'U'; 'W'; 'X'; 'Y'; 'Z']  outPortNames=['v'; 'c'; '0'; '1'; '2'; '3'; '4'; '5'; '6'; '7'; '8'; '9'; 'A'; 'B'; 'D'; 'E'; 'F'; 'G'; 'H'; 'I'; 'J'; 'K'; 'L'; 'M'; 'N'; 'O'; 'P'; 'Q'; 'R'; 'S'; 'T'; 'U'; 'W'; 'X'; 'Y'; 'Z']  dspbaimage=dspba_prim.jpg  text=fprintf('In');  style=Optimised  dataSignals=4  foldingEnabled=off  channels=1  sampleRate=200  packetBeginPresent=off  packetBeginEnabled=off  visibilities=dspba_ChannelInVis(gcb)  latencyCorrection=0  version=20141013
  ChannelOut : DSPBAPrim/ChannelOut  primtype=channelout  nInputs=dspba_internal_get_channel_ports(gcb)  nOutputs=dspba_internal_get_channel_ports(gcb)  omode=Inherit via internal rule  otype=sfix(16)  scale=2^-15  rndmethod=Unbiased  factor=1  satmethod=Symmetric  shift_vec=[0 1 2 -1]  value=13  inPortNames=['v'; 'c'; '0'; '1'; '2'; '3'; '4'; '5'; '6'; '7'; '8'; '9'; 'A'; 'B'; 'D'; 'E'; 'F'; 'G'; 'H'; 'I'; 'J'; 'K'; 'L'; 'M'; 'N'; 'O'; 'P'; 'Q'; 'R'; 'S'; 'T'; 'U'; 'W'; 'X'; 'Y'; 'Z']  outPortNames=['v'; 'c'; '0'; '1'; '2'; '3'; '4'; '5'; '6'; '7'; '8'; '9'; 'A'; 'B'; 'D'; 'E'; 'F'; 'G'; 'H'; 'I'; 'J'; 'K'; 'L'; 'M'; 'N'; 'O'; 'P'; 'Q'; 'R'; 'S'; 'T'; 'U'; 'W'; 'X'; 'Y'; 'Z']  dspbaimage=dspba_prim.jpg  text=fprintf('Out%s', AdvDSPBChannelOutDisplay(latency));  style=Optimised  dataSignals=13  foldingEnabled=off  channels=1  sampleRate=200  packetBeginPresent=off  packetBeginEnabled=off  visibilities=dspba_ChannelOutVis(gcb)  latency=7  latencyCorrection=0  version=20141013
  Const{,1..25} (26 alike) : DSPBAPrim/Const  primtype=const  nInputs=0  nOutputs=1  omode=single  otype=sfix(16)  scale=2^-15  rndmethod=Unbiased  factor=1  satmethod=Symmetric  shift_vec=[0 1 2 -1]  value=0  inPortNames=['+'; '+';]  outPortNames=[' ']  dspbaimage=dspba_prim.jpg  text=fprintf('%s', num2str(value));  style=Optimised  visibilities=8 + 1024  floatPrecision=float32_m23  version=20120820
  MultAcc{,1..12} (13 alike) : DSPBAPrim/MultAcc  primtype=multaccfunc  nInputs=3  nOutputs=1  omode=Inherit via internal rule  otype=sfix(16)  scale=2^-15  rndmethod=Unbiased  factor=1  satmethod=Symmetric  shift_vec=[0 1 2 -1]  value=0  inPortNames="[ 'acc'; 'x  '; 'y  ']"  outPortNames=[]  dspbaimage=dspba_prim_float.jpg  text=disp('multAcc');  style=Optimised  visibilities=8+2^17  functionExpr=fpMultAcc  advOptions=[]  version=20121130
  Mux{,1..25} (26 alike) : DSPBAPrim/Mux  primtype=mux  nInputs=evalAionMaskParam(gcb,'value',1)+1  nOutputs=1  omode=Inherit via internal rule  otype=sfix(16)  scale=2^-15  rndmethod=Unbiased  factor=1  satmethod=Symmetric  shift_vec=[0 1 2 -1]  value=2  inPortNames=['s '; 'd0'; 'd1'; 'd2'; 'd3'; 'd4'; 'd5'; 'd6'; 'd7'; 'd8'; 'd9';]  outPortNames=[' ']  dspbaimage=dspba_prim.jpg  text=fprintf('%s', primtype);  style=Optimised  visibilities=1032  version=20131025
  Not : DSPBAPrim/Not  primtype=not  nInputs=1  nOutputs=1  omode=Inherit via internal rule  otype=sfix(16)  scale=2^-15  rndmethod=Unbiased  factor=1  satmethod=Symmetric  shift_vec=[0 1 2 -1]  value=0  inPortNames=[' '; ' ';]  outPortNames=[' ']  dspbaimage=dspba_prim.jpg  text=fprintf('~');  style=Optimised  visibilities=8  version=20090407
  Or : DSPBAPrim/Or  primtype=or  nInputs=2  nOutputs=1  omode=Inherit via internal rule  otype=sfix(16)  scale=2^-15  rndmethod=Unbiased  factor=1  satmethod=Symmetric  shift_vec=[0 1 2 -1]  value=0  inPortNames=[' '; ' '; ' '; ' '; ' '; ' '; ' '; ' '; ' '; ' '; ' '; ' '; ' '; ' '; ' '; ' '; ]  outPortNames=[' ']  dspbaimage=dspba_prim.jpg  text=fprintf('|');  style=Optimised  visibilities=8+2  version=20090407
  SampleDelay{,1..36,38} (38 alike) : DSPBAPrim/SampleDelay  primtype=sampdelay  nInputs=1  nOutputs=1  omode=Inherit via internal rule  otype=sfix(16)  scale=2^-15  rndmethod=Unbiased  factor=1  satmethod=Symmetric  shift_vec=[0 1 2 -1]  value=1  inPortNames=[' '; ' ';]  outPortNames=[' ']  dspbaimage=dspba_prim.jpg  text=dpoly(1, eye(1,value+1), 'z')  style=Optimised  visibilities=8 + 1024 + 2^17 + 2^18  flexible=off  slackgroup=0  augmented=0  version=20090407  advOptions=[]
  Scope1 : Scope  NumInputPorts=4
  Scope2 : Scope  NumInputPorts=4
  Scope3 : Scope  NumInputPorts=4
  SynthesisInfo : DSPBAPrim/SynthesisInfo  primtype=synthinfo  nInputs=0  nOutputs=0  omode=Inherit via internal rule  otype=sfix(16)  scale=2^-15  rndmethod=Truncate  factor=1  satmethod=Symmetric  shift_vec=[0 1 2 -1]  value=99  inPortNames=[' '; ' ';]  outPortNames=[' ']  dspbaimage=dspba_prim_ctrl.jpg  text=fprintf('Style=%s', style);  style=Scheduled  visibilities=2^15+2^17+2^18+2^19  constraintInUse=on  constraintRelation==  constraintLimit=7  bitAccurate=off  version=20150220
  single_delay : Subsystem  Commented=on
  vout : Outport
  cout : Outport  Port=2
  M0 : Outport  Port=3
  M1 : Outport  Port=4
  M2 : Outport  Port=5
  M3 : Outport  Port=6
  M4 : Outport  Port=7
  M5 : Outport  Port=8
  M6 : Outport  Port=9
  M7 : Outport  Port=10
  M8 : Outport  Port=11
  M9 : Outport  Port=12
  M10 : Outport  Port=13
  M11 : Outport  Port=14
  M12 : Outport  Port=15
  wires:
  ChannelIn/4 -> Mux12/3, Scope2/2
  ChannelIn/3 -> SampleDelay38/1
  Mux1/1 -> SampleDelay/1
  Mux2/1 -> SampleDelay1/1
  Mux3/1 -> SampleDelay2/1
  Mux4/1 -> SampleDelay3/1
  Mux5/1 -> SampleDelay4/1
  Mux6/1 -> SampleDelay5/1
  Mux7/1 -> SampleDelay6/1
  Mux8/1 -> SampleDelay7/1
  Mux9/1 -> SampleDelay8/1
  Mux10/1 -> SampleDelay9/1
  Mux11/1 -> SampleDelay10/1
  valid/1 -> ChannelIn/1  "qv"
  channel/1 -> ChannelIn/2  "qc"
  Ai/1 -> ChannelIn/3
  Bi-Bq/1 -> ChannelIn/4
  Acc_clear/1 -> ChannelIn/5
  ChannelOut/1 -> vout/1
  ChannelOut/2 -> cout/1
  ChannelOut/3 -> M0/1
  ChannelOut/4 -> M1/1
  ChannelOut/5 -> M2/1
  ChannelOut/6 -> M3/1
  ChannelOut/7 -> M4/1
  ChannelOut/8 -> M5/1
  ChannelOut/9 -> M6/1
  ChannelOut/10 -> M7/1
  ChannelOut/11 -> M8/1
  ChannelOut/12 -> M9/1
  ChannelOut/13 -> M10/1
  ChannelOut/14 -> M11/1
  ChannelOut/15 -> M12/1
  MultAcc/1 -> ChannelOut/3
  MultAcc1/1 -> ChannelOut/4
  MultAcc2/1 -> ChannelOut/5
  MultAcc3/1 -> ChannelOut/6
  MultAcc4/1 -> ChannelOut/7
  MultAcc5/1 -> ChannelOut/8
  MultAcc6/1 -> ChannelOut/9
  MultAcc7/1 -> ChannelOut/10
  MultAcc8/1 -> ChannelOut/11
  MultAcc9/1 -> ChannelOut/12
  MultAcc10/1 -> ChannelOut/13
  MultAcc11/1 -> ChannelOut/14
  MultAcc12/1 -> ChannelOut/15
  ChannelIn/1 -> Mux12/1, SampleDelay12/1, Scope2/1  "qv"
  ChannelIn/2 -> ChannelOut/2  "qc"
  SampleDelay24/1 -> Mux13/3, Scope2/4, Scope3/2, Mux/3
  SampleDelay11/1 -> Scope3/4, Mux14/3, Scope1/2, Mux1/3
  SampleDelay/1 -> Mux15/3, Scope1/4, Mux2/3
  SampleDelay1/1 -> Mux16/3, Mux3/3
  SampleDelay2/1 -> Mux17/3, Mux4/3
  SampleDelay3/1 -> Mux18/3, Mux5/3
  SampleDelay4/1 -> Mux19/3, Mux6/3
  SampleDelay6/1 -> Mux21/3, Mux8/3
  SampleDelay7/1 -> Mux22/3, Mux9/3
  SampleDelay9/1 -> Mux24/3, Mux11/3
  Const/1 -> Mux/2
  Const1/1 -> Mux1/2
  Const2/1 -> Mux2/2
  Const3/1 -> Mux3/2
  Const4/1 -> Mux4/2
  Const5/1 -> Mux5/2
  Const6/1 -> Mux6/2
  Const7/1 -> Mux7/2
  Const8/1 -> Mux8/2
  Const9/1 -> Mux9/2
  Const10/1 -> Mux10/2
  Const11/1 -> Mux11/2
  SampleDelay5/1 -> Mux20/3, Mux7/3
  SampleDelay8/1 -> Mux23/3, Mux10/3
  SampleDelay10/1 -> Mux25/3
  Mux/1 -> SampleDelay11/1
  ChannelIn/5 -> Or/2
  ChannelIn/6 -> Or/1
  SOP_in/1 -> ChannelIn/6
  SampleDelay12/1 -> SampleDelay13/1, Scope3/1, Mux/1
  SampleDelay13/1 -> SampleDelay14/1, Scope1/1, Mux1/1
  SampleDelay14/1 -> SampleDelay15/1, Mux2/1
  SampleDelay15/1 -> SampleDelay16/1, Mux3/1
  SampleDelay16/1 -> SampleDelay17/1, Mux4/1
  SampleDelay17/1 -> SampleDelay18/1, Mux5/1
  SampleDelay18/1 -> SampleDelay19/1, Mux6/1
  SampleDelay19/1 -> SampleDelay20/1, Mux7/1
  SampleDelay20/1 -> SampleDelay21/1, Mux8/1
  SampleDelay21/1 -> SampleDelay22/1, Mux9/1
  SampleDelay22/1 -> SampleDelay23/1, Mux10/1
  SampleDelay23/1 -> ChannelOut/1, Mux11/1
  SampleDelay25/1 -> Mux14/1, MultAcc1/1, SampleDelay26/1
  SampleDelay26/1 -> MultAcc2/1, Mux15/1, SampleDelay27/1
  SampleDelay27/1 -> MultAcc3/1, Mux16/1, SampleDelay28/1
  SampleDelay28/1 -> Mux17/1, MultAcc4/1, SampleDelay29/1
  SampleDelay29/1 -> Mux18/1, MultAcc5/1, SampleDelay30/1
  SampleDelay30/1 -> MultAcc6/1, Mux19/1, SampleDelay31/1
  SampleDelay31/1 -> MultAcc7/1, Mux20/1, SampleDelay32/1
  SampleDelay32/1 -> MultAcc8/1, Mux21/1, SampleDelay33/1
  SampleDelay33/1 -> MultAcc9/1, Mux22/1, SampleDelay34/1
  SampleDelay34/1 -> MultAcc10/1, Mux23/1, SampleDelay35/1
  SampleDelay35/1 -> MultAcc11/1, Mux24/1, SampleDelay36/1
  SampleDelay36/1 -> MultAcc12/1, Mux25/1
  Const12/1 -> Mux12/2
  Mux12/1 -> SampleDelay24/1
  SampleDelay38/1 -> Scope2/3, MultAcc/3, Scope3/3, MultAcc1/3, Scope1/3, MultAcc2/3, MultAcc3/3, MultAcc5/3, MultAcc8/3, MultAcc9/3, MultAcc12/3, MultAcc11/3, MultAcc10/3, MultAcc7/3, MultAcc6/3, MultAcc4/3
  Or/1 -> Not/1
  Mux13/1 -> MultAcc/2
  Not/1 -> Mux13/1, MultAcc/1, SampleDelay25/1
  Const13/1 -> Mux13/2
  Const14/1 -> Mux14/2
  Mux14/1 -> MultAcc1/2
  Const15/1 -> Mux15/2
  Mux15/1 -> MultAcc2/2
  Const16/1 -> Mux16/2
  Mux16/1 -> MultAcc3/2
  Const17/1 -> Mux17/2
  Mux17/1 -> MultAcc4/2
  Const18/1 -> Mux18/2
  Mux18/1 -> MultAcc5/2
  Const19/1 -> Mux19/2
  Mux19/1 -> MultAcc6/2
  Const20/1 -> Mux20/2
  Mux20/1 -> MultAcc7/2
  Const21/1 -> Mux21/2
  Mux21/1 -> MultAcc8/2
  Const22/1 -> Mux22/2
  Mux22/1 -> MultAcc9/2
  Const23/1 -> Mux23/2
  Mux23/1 -> MultAcc10/2
  Const24/1 -> Mux24/2
  Mux24/1 -> MultAcc11/2
  Const25/1 -> Mux25/2
  Mux25/1 -> MultAcc12/2
